simulink model "Prob1a"  (Simulink 7.0)
settings: Solver=ode45  StartTime=0.0  StopTime=10.0  RelTol=1e-3
settings Model: Creator=Kailu  LastModifiedBy=Kailu

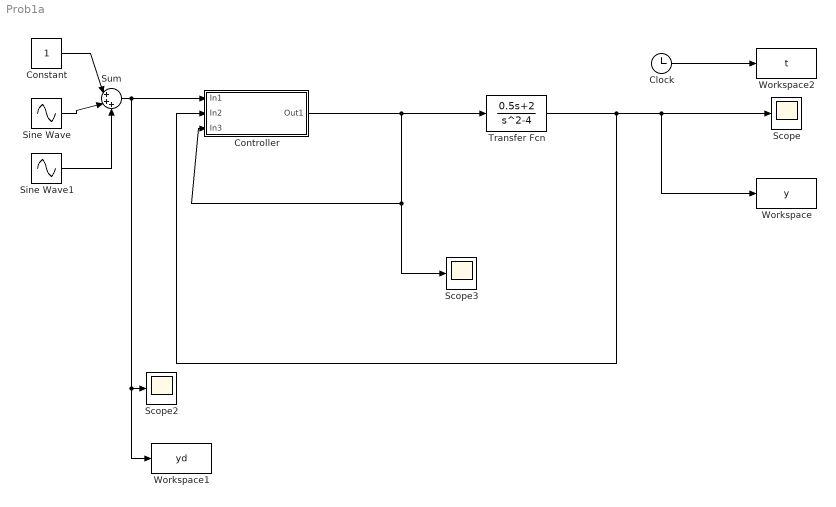
== system Prob1a ==
  Clock : Clock
      settings: Decimation=10
  Constant : Constant  OutDataType=sfix(16)  OutScaling=2^0
  Controller : Subsystem
  Scope : Scope
  Scope2 : Scope
      settings: SaveName=ScopeData2
  Scope3 : Scope
      settings: SaveName=ScopeData3
  Sine Wave : Sin  SampleTime=0
  Sine Wave1 : Sin  Frequency=2  SampleTime=0
  Sum : Sum  Inputs=|+++  OutDataType=sfix(16)  OutScaling=2^0
  Transfer Fcn : TransferFcn  Numerator=[ 0.5 2]  Denominator=[1 0 -4]
  Workspace : ToWorkspace  VariableName=y  SampleTime=-1  SaveFormat=Array
  Workspace1 : ToWorkspace  VariableName=yd  SampleTime=-1  SaveFormat=Array
  Workspace2 : ToWorkspace  VariableName=t  SampleTime=-1  SaveFormat=Array
  wires:
  Controller/1(Out1) -> Transfer Fcn/1, Controller/3(In3), Scope3/1
  Transfer Fcn/1 -> Controller/2(In2), Scope/1, Workspace/1
  Constant/1 -> Sum/1
  Sine Wave/1 -> Sum/2
  Sine Wave1/1 -> Sum/3
  Sum/1 -> Controller/1(In1), Scope2/1, Workspace1/1
  Clock/1 -> Workspace2/1

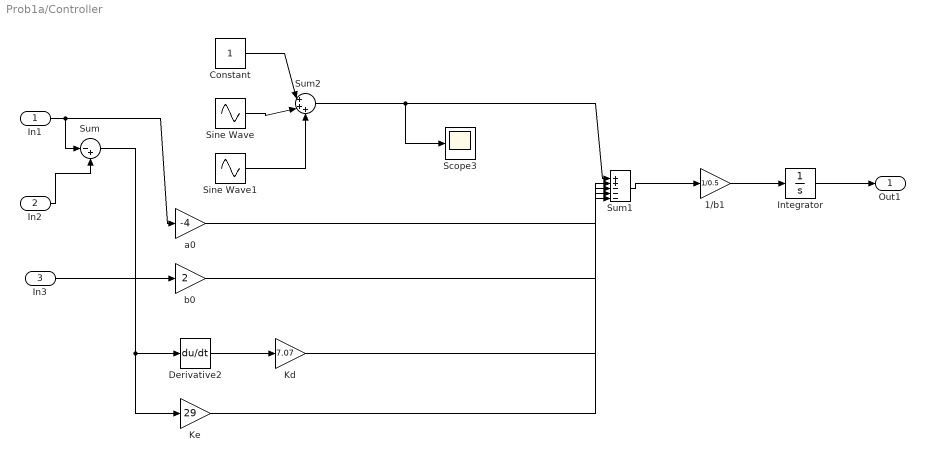
== system Prob1a/Controller ==
  In1 : Inport  OutDataType=sfix(16)  OutScaling=2^0
  In2 : Inport  Port=2  OutDataType=sfix(16)  OutScaling=2^0
  In3 : Inport  Port=3  OutDataType=sfix(16)  OutScaling=2^0
  1/b1 : Gain  Gain=1/0.5  ParameterDataType=sfix(16)  ParameterScaling=2^0  OutDataType=sfix(16)  OutScaling=2^0
  Constant : Constant  OutDataType=sfix(16)  OutScaling=2^0
  Derivative2 : Derivative
  Integrator : Integrator
  Kd : Gain  Gain=7.07  ParameterDataType=sfix(16)  ParameterScaling=2^0  OutDataType=sfix(16)  OutScaling=2^0
  Ke : Gain  Gain=29  ParameterDataType=sfix(16)  ParameterScaling=2^0  OutDataType=sfix(16)  OutScaling=2^0
  Scope3 : Scope
      settings: SaveName=ScopeData4
  Sine Wave : Sin  Amplitude=-1  SampleTime=0
  Sine Wave1 : Sin  Amplitude=-4  Frequency=2  SampleTime=0
  Sum : Sum  Inputs=|-+  OutDataType=sfix(16)  OutScaling=2^0
  Sum1 : Sum  Inputs=|++---  OutDataType=sfix(16)  OutScaling=2^0
  Sum2 : Sum  Inputs=|+++  OutDataType=sfix(16)  OutScaling=2^0
  a0 : Gain  Gain=-4  ParameterDataType=sfix(16)  ParameterScaling=2^0  OutDataType=sfix(16)  OutScaling=2^0
  b0 : Gain  Gain=2  ParameterDataType=sfix(16)  ParameterScaling=2^0  OutDataType=sfix(16)  OutScaling=2^0
  Out1 : Outport  OutDataType=sfix(16)  OutScaling=2^0
  wires:
  1/b1/1 -> Integrator/1
  Integrator/1 -> Out1/1
  In2/1 -> Sum/2
  a0/1 -> Sum1/2
  In3/1 -> b0/1
  b0/1 -> Sum1/3
  In1/1 -> Sum/1, a0/1
  Sum/1 -> Derivative2/1, Ke/1
  Derivative2/1 -> Kd/1
  Kd/1 -> Sum1/4
  Ke/1 -> Sum1/5
  Sum1/1 -> 1/b1/1
  Constant/1 -> Sum2/1
  Sine Wave/1 -> Sum2/2
  Sine Wave1/1 -> Sum2/3
  Sum2/1 -> Sum1/1, Scope3/1
